simulink model "CONT_MOD"  (Simulink 5.0)
settings: Solver=ode45  StartTime=0.0  StopTime=10.0  RelTol=1e-3
settings Model: LastModifiedBy=Administrator

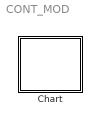
== system CONT_MOD ==
  Chart : Stateflow chart

== stateflow chart Chart ==
  state A/
    state A1/
      state A11/
        during:
      state A12/
      (default) -> A11 : [1]
      A12 -> A11 : [IV>0]
      A11 -> A12 : [IV<=0]
    state A2/
      during:Q6=1;Q5=1;Q1=0;Q2=0;
      Q3=0;Q4=0;
    A1 -> A2 : [IV>IVSTAR]
    A2 -> A1 : [IV<IVSTAR]
